simulink model "SYSTEM"  (R2026a)
settings: Solver=VariableStepAuto
model workspace (MAT data in the model file):
  CompAir_P : Simulink.ConnectionBus (value not decoded)
  CompAir_S : Simulink.Bus (value not decoded)
  Control_P : Simulink.ConnectionBus (value not decoded)
  Control_S : Simulink.Bus (value not decoded)
  CoolingFW_P : Simulink.ConnectionBus (value not decoded)
  CoolingFW_S : Simulink.Bus (value not decoded)
  FuelOil_P : Simulink.ConnectionBus (value not decoded)
  FuelOil_S : Simulink.Bus (value not decoded)
  Heat_P : Simulink.ConnectionBus (value not decoded)
  Heat_S : Simulink.Bus (value not decoded)
  LubeOil_P : Simulink.ConnectionBus (value not decoded)
  LubeOil_S : Simulink.Bus (value not decoded)
  Physical : Simulink.ConnectionBus (value not decoded)
  Power_P : Simulink.ConnectionBus (value not decoded)
  Power_S : Simulink.Bus (value not decoded)
  SaltWater_P : Simulink.ConnectionBus (value not decoded)
  SaltWater_S : Simulink.Bus (value not decoded)
  WasteGas_P : Simulink.ConnectionBus (value not decoded)
  WasteGas_S : Simulink.Bus (value not decoded)
  WasteOil_P : Simulink.ConnectionBus (value not decoded)
  WasteOil_S : Simulink.Bus (value not decoded)
  WasteSolid_P : Simulink.ConnectionBus (value not decoded)
  WasteSolid_S : Simulink.Bus (value not decoded)
  WasteWater_P : Simulink.ConnectionBus (value not decoded)
  WasteWater_S : Simulink.Bus (value not decoded)
undefined symbols (not defined in the file): FUEL
(part 5 of 5)

== system SYSTEM/SHIP/200 (PROPULSION)/21X (PROPULSORS)/21X WATER JET + MANEUVERING THRUSTER ==
  Bus Element In1 : Inport  PortName=42X-21XC
  Bus Element In3 : Inport  Port=2  PortName=51X-21XLO
  Bus Element In4 : Inport  Port=3  PortName=53X-21XCA
  Bus Element In2 : Inport  Port=4  PortName=50X-21XCFW
  10X-21X : PMIOPort  Side=Right  ConnectionType=Bus: Physical
  FROM 22X : PMIOPort  Port=2  Side=Right  ConnectionType=Bus: Physical
  Bus Element Out1 : Outport  PortName=21X-42XC
  Bus Element Out3 : Outport  Port=2  PortName=21X-51XLO
  Bus Element Out4 : Outport  Port=3  PortName=21X-53XCA
  Bus Element Out2 : Outport  Port=4  PortName=21X-50XCFW

== system SYSTEM/SHIP/200 (PROPULSION)/22X (SHAFTING)/22X ABSENT ==

== system SYSTEM/SHIP/200 (PROPULSION)/22X (SHAFTING)/22X MECHANICAL ==
  Bus Element In1 : Inport  PortName=51X-22XLO
  Bus Element In2 : Inport  Port=2  PortName=53X-22XCA
  TOFROM 23X : PMIOPort  Side=Right  ConnectionType=Bus: Physical
  10X-22X : PMIOPort  Port=2  Side=Right  ConnectionType=Bus: Physical
  TO 21X : PMIOPort  Port=3  Side=Right  ConnectionType=Bus: Physical
  Bus Element Out2 : Outport  PortName=22X-51XLO
  Bus Element Out3 : Outport  Port=2  PortName=22X-53XCA
  Bus Element Out1 : Outport  Port=3  PortName=22X-42XC

== system SYSTEM/SHIP/200 (PROPULSION)/23X (POWER TRANSMISSION)/23X ABSENT ==

== system SYSTEM/SHIP/200 (PROPULSION)/23X (POWER TRANSMISSION)/23X MECHANICAL ==
  Bus Element In2 : Inport  PortName=51X-23XLO
  Bus Element In1 : Inport  Port=2  PortName=42X-23XC
  TOFROM 22X : PMIOPort  Side=Left  ConnectionType=Bus: Physical
  FROM 20X : PMIOPort  Port=2  Side=Left  ConnectionType=Bus: Physical
  10X-23X : PMIOPort  Port=3  Side=Right  ConnectionType=Bus: Physical
  Bus Element Out3 : Outport  PortName=23X-51XLO
  Bus Element Out2 : Outport  Port=2  PortName=23X-42XC
  Bus Element Out1 : Outport  Port=3  PortName=23X-31XP

== system SYSTEM/SHIP/200 (PROPULSION)/23X (POWER TRANSMISSION)/23X MECHANICAL WITH POWER TAKEOFF ==
  Bus Element In2 : Inport  PortName=51X-23XLO
  Bus Element In1 : Inport  Port=2  PortName=42X-23XC
  TOFROM 22X : PMIOPort  Side=Left  ConnectionType=Bus: Physical
  FROM 20X : PMIOPort  Port=2  Side=Left  ConnectionType=Bus: Physical
  10X-23X : PMIOPort  Port=3  Side=Right  ConnectionType=Bus: Physical
  Bus Element Out3 : Outport  PortName=23X-51XLO
  Bus Element Out2 : Outport  Port=2  PortName=23X-42XC
  Bus Element Out1 : Outport  Port=3  PortName=23X-31XP

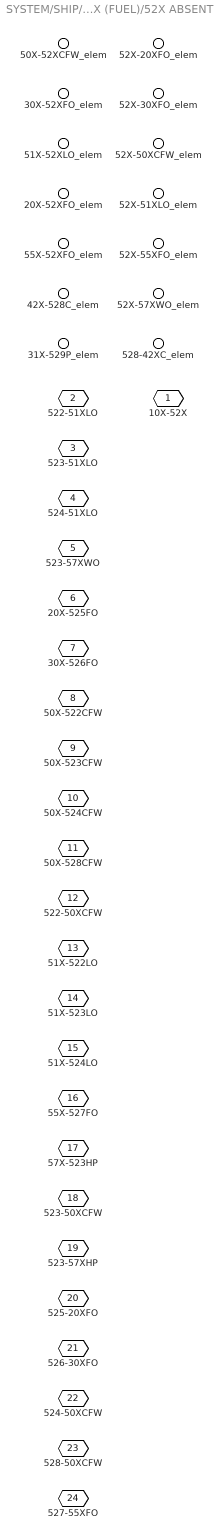
== system SYSTEM/SHIP/500 (AUXILLIARY SYSTEMS)/52X (FUEL)/52X ABSENT ==
  50X-52XCFW_elem : Inport  PortName=50X-52XCFW
  30X-52XFO_elem : Inport  Port=2  PortName=30X-52XFO
  51X-52XLO_elem : Inport  Port=3  PortName=51X-52XLO
  20X-52XFO_elem : Inport  Port=4  PortName=20X-52XFO
  55X-52XFO_elem : Inport  Port=5  PortName=55X-52XFO
  42X-528C_elem : Inport  Port=6  PortName=42X-528C
  31X-529P_elem : Inport  Port=7  PortName=31X-529P
  10X-52X : PMIOPort  Side=Right
  522-51XLO : PMIOPort  Port=2  Side=Left  ConnectionType=Bus: LubeOil_P
  523-51XLO : PMIOPort  Port=3  Side=Left  ConnectionType=Bus: LubeOil_P
  524-51XLO : PMIOPort  Port=4  Side=Left  ConnectionType=Bus: LubeOil_P
  523-57XWO : PMIOPort  Port=5  Side=Left  ConnectionType=Bus: WasteOil_P
  20X-525FO : PMIOPort  Port=6  Side=Left  ConnectionType=Bus: FuelOil_P
  30X-526FO : PMIOPort  Port=7  Side=Left  ConnectionType=Bus: FuelOil_P
  50X-522CFW : PMIOPort  Port=8  Side=Left  ConnectionType=Bus: CoolingFW_P
  50X-523CFW : PMIOPort  Port=9  Side=Left  ConnectionType=Bus: CoolingFW_P
  50X-524CFW : PMIOPort  Port=10  Side=Left  ConnectionType=Bus: CoolingFW_P
  50X-528CFW : PMIOPort  Port=11  Side=Left  ConnectionType=Bus: CoolingFW_P
  522-50XCFW : PMIOPort  Port=12  Side=Left  ConnectionType=Bus: CoolingFW_P
  51X-522LO : PMIOPort  Port=13  Side=Left  ConnectionType=Bus: LubeOil_P
  51X-523LO : PMIOPort  Port=14  Side=Left  ConnectionType=Bus: LubeOil_P
  51X-524LO : PMIOPort  Port=15  Side=Left  ConnectionType=Bus: LubeOil_P
  55X-527FO : PMIOPort  Port=16  Side=Left  ConnectionType=Bus: FuelOil_P
  57X-523HP : PMIOPort  Port=17  Side=Left  ConnectionType=Bus: Heat_P
  523-50XCFW : PMIOPort  Port=18  Side=Left  ConnectionType=Bus: CoolingFW_P
  523-57XHP : PMIOPort  Port=19  Side=Left  ConnectionType=Bus: Heat_P
  525-20XFO : PMIOPort  Port=20  Side=Left  ConnectionType=Bus: FuelOil_P
  526-30XFO : PMIOPort  Port=21  Side=Left  ConnectionType=Bus: FuelOil_P
  524-50XCFW : PMIOPort  Port=22  Side=Left  ConnectionType=Bus: CoolingFW_P
  528-50XCFW : PMIOPort  Port=23  Side=Left  ConnectionType=Bus: CoolingFW_P
  527-55XFO : PMIOPort  Port=24  Side=Left  ConnectionType=Bus: FuelOil_P
  52X-20XFO_elem : Outport  PortName=52X-20XFO
  52X-30XFO_elem : Outport  Port=2  PortName=52X-30XFO
  52X-50XCFW_elem : Outport  Port=3  PortName=52X-50XCFW
  52X-51XLO_elem : Outport  Port=4  PortName=52X-51XLO
  52X-55XFO_elem : Outport  Port=5  PortName=52X-55XFO
  52X-57XWO_elem : Outport  Port=6  PortName=52X-57XWO
  528-42XC_elem : Outport  Port=7  PortName=528-42XC

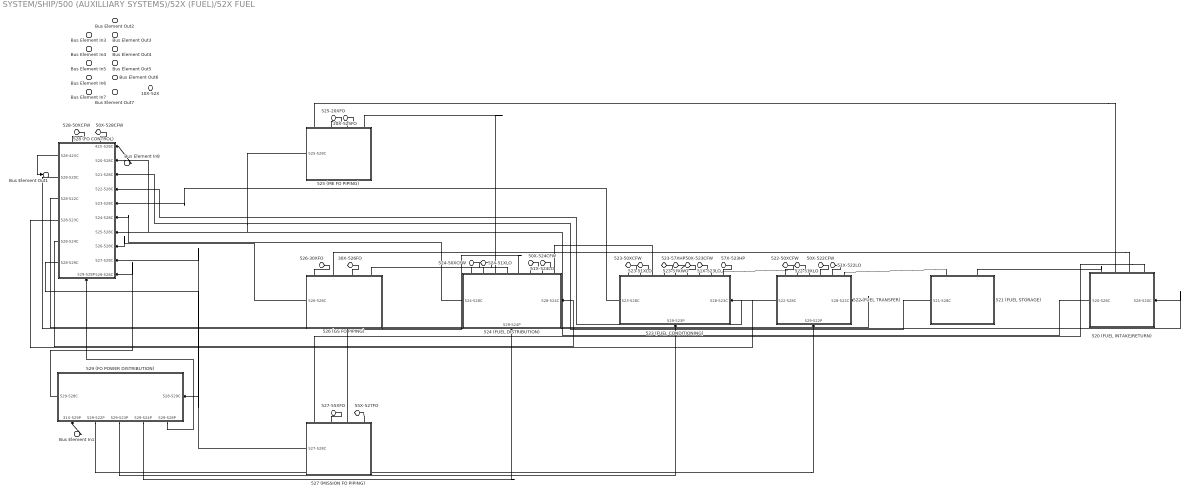
== system SYSTEM/SHIP/500 (AUXILLIARY SYSTEMS)/52X (FUEL)/52X FUEL ==
  Bus Element In3 : Inport  PortName=50X-52XCFW
  Bus Element In6 : Inport  Port=2  PortName=30X-52XFO
  Bus Element In4 : Inport  Port=3  PortName=51X-52XLO
  Bus Element In5 : Inport  Port=4  PortName=20X-52XFO
  Bus Element In7 : Inport  Port=5  PortName=55X-52XFO
  Bus Element In8 : Inport  Port=6  PortName=42X-528C
  Bus Element In1 : Inport  Port=7  PortName=31X-529P
  520 (FUEL INTAKE/RETURN) : Subsystem
      settings: PortSchema="{\"entries\":[{\"content\":{\"headerSize\":26,\"margin\":15,\"minimumSpacing\":25,\"sides\":[{\"content\":{\"connectorIds\":[\"Out1\"]},\"type\":\"ConnectorPlacement.EquallySpacedRectSide\",\"uuid\":\"4cfdffe2-3a28-4674-9aac-ff2f96812f2a\"},{\"content\":{\"connectorIds\":[\"In1\"],\"side\":\"RIGHT\"},\"type\":\"ConnectorPlacement.EquallySpacedRectSide\",\"uuid\":\"6bc321b8-6efb-4233-b1c1-d1363ffaceac\"},{\"content\":{\"connectorIds\":[\"LConn1\",\"RConn1\",\"RConn2\",\"RConn3\"],\"side\":\"TOP\"},\"type\":\"ConnectorPlacement.EquallySpacedRectSide\",\"uuid\":\"5128f762-77ab-4823-b460-d8c60ef20dad\"}]},\"type\":\"ConnectorPlacement.EquallySpacedConnector\",\"uuid\":\"2fe14ae3-6aef-4ed5-a4dc-a282704d28f8\"}],\"packageUris\":[\"http://schema.mathworks.com/mf0/Connector/R2020b\"],\"version\":\"1.0\"}"
  521 (FUEL STORAGE) : Subsystem
      settings: PortSchema="{\"entries\":[{\"content\":{\"headerSize\":26,\"margin\":15,\"minimumSpacing\":25,\"sides\":[{\"content\":{\"connectorIds\":[\"Out1\"]},\"type\":\"ConnectorPlacement.EquallySpacedRectSide\",\"uuid\":\"4cfdffe2-3a28-4674-9aac-ff2f96812f2a\"},{\"content\":{\"side\":\"RIGHT\"},\"type\":\"ConnectorPlacement.EquallySpacedRectSide\",\"uuid\":\"6bc321b8-6efb-4233-b1c1-d1363ffaceac\"},{\"content\":{\"connectorIds\":[\"LConn1\",\"RConn1\"],\"side\":\"TOP\"},\"type\":\"ConnectorPlacement.EquallySpacedRectSide\",\"uuid\":\"5128f762-77ab-4823-b460-d8c60ef20dad\"}]},\"type\":\"ConnectorPlacement.EquallySpacedConnector\",\"uuid\":\"2fe14ae3-6aef-4ed5-a4dc-a282704d28f8\"}],\"packageUris\":[\"http://schema.mathworks.com/mf0/Connector/R2020b\"],\"version\":\"1.0\"}"
  522 (FUEL TRANSFER) : Subsystem
      settings: PortSchema="{\"entries\":[{\"content\":{\"headerSize\":26,\"margin\":15,\"minimumSpacing\":25,\"sides\":[{\"content\":{\"connectorIds\":[\"Out1\"]},\"type\":\"ConnectorPlacement.EquallySpacedRectSide\",\"uuid\":\"4cfdffe2-3a28-4674-9aac-ff2f96812f2a\"},{\"content\":{\"connectorIds\":[\"In2\"],\"side\":\"RIGHT\"},\"type\":\"ConnectorPlacement.EquallySpacedRectSide\",\"uuid\":\"6bc321b8-6efb-4233-b1c1-d1363ffaceac\"},{\"content\":{\"connectorIds\":[\"LConn3\",\"LConn2\",\"LConn1\",\"LConn4\",\"LConn5\",\"RConn1\"],\"side\":\"TOP\"},\"type\":\"ConnectorPlacement.EquallySpacedRectSide\",\"uuid\":\"5128f762-77ab-4823-b460-d8c60ef20dad\"},{\"content\":{\"connectorIds\":[\"In1\"],\"side\":\"BOTTOM\"},\"type\":\"ConnectorPlacement.EquallySpacedRectSide\",\"uuid\":\"2a930d33-7a6a-4e0b-9580-44c950610589\"}]},\"type\":\"ConnectorPlacement.EquallySpacedConnector\",\"uuid\":\"2fe14ae3-6aef-4ed5-a4dc-a282704d28f8\"}],\"packageUris\":[\"http://schema.mathworks.com/mf0/Connector/R2020b\"],\"version\":\"1.0\"}"
  523 (FUEL CONDITIONING) : Subsystem
      settings: PortSchema="{\"entries\":[{\"content\":{\"headerSize\":26,\"margin\":15,\"minimumSpacing\":25,\"sides\":[{\"content\":{\"connectorIds\":[\"Out1\"]},\"type\":\"ConnectorPlacement.EquallySpacedRectSide\",\"uuid\":\"4cfdffe2-3a28-4674-9aac-ff2f96812f2a\"},{\"content\":{\"connectorIds\":[\"In2\"],\"side\":\"RIGHT\"},\"type\":\"ConnectorPlacement.EquallySpacedRectSide\",\"uuid\":\"6bc321b8-6efb-4233-b1c1-d1363ffaceac\"},{\"content\":{\"connectorIds\":[\"LConn3\",\"LConn2\",\"LConn1\",\"RConn2\",\"LConn4\",\"LConn5\",\"LConn6\",\"RConn3\",\"RConn1\"],\"side\":\"TOP\"},\"type\":\"ConnectorPlacement.EquallySpacedRectSide\",\"uuid\":\"5128f762-77ab-4823-b460-d8c60ef20dad\"},{\"content\":{\"connectorIds\":[\"In1\"],\"side\":\"BOTTOM\"},\"type\":\"ConnectorPlacement.EquallySpacedRectSide\",\"uuid\":\"0a36b159-1b21-43db-be33-33362cd12218\"}]},\"type\":\"ConnectorPlacement.EquallySpacedConnector\",\"uuid\":\"2fe14ae3-6aef-4ed5-a4dc-a282704d28f8\"}],\"packageUris\":[\"http://schema.mathworks.com/mf0/Connector/R2020b\"],\"version\":\"1.0\"}"
  524 (FUEL DISTRIBUTION) : Subsystem
      settings: PortSchema="{\"entries\":[{\"content\":{\"headerSize\":26,\"margin\":15,\"minimumSpacing\":25,\"sides\":[{\"content\":{\"connectorIds\":[\"Out1\"]},\"type\":\"ConnectorPlacement.EquallySpacedRectSide\",\"uuid\":\"4cfdffe2-3a28-4674-9aac-ff2f96812f2a\"},{\"content\":{\"connectorIds\":[\"In2\"],\"side\":\"RIGHT\"},\"type\":\"ConnectorPlacement.EquallySpacedRectSide\",\"uuid\":\"6bc321b8-6efb-4233-b1c1-d1363ffaceac\"},{\"content\":{\"connectorIds\":[\"LConn5\",\"LConn2\",\"LConn1\",\"LConn3\",\"LConn4\",\"LConn6\",\"LConn7\",\"RConn1\"],\"side\":\"TOP\"},\"type\":\"ConnectorPlacement.EquallySpacedRectSide\",\"uuid\":\"5128f762-77ab-4823-b460-d8c60ef20dad\"},{\"content\":{\"connectorIds\":[\"In1\"],\"side\":\"BOTTOM\"},\"type\":\"ConnectorPlacement.EquallySpacedRectSide\",\"uuid\":\"af17bfb2-26c0-4d79-9f41-99ac55d94094\"}]},\"type\":\"ConnectorPlacement.EquallySpacedConnector\",\"uuid\":\"2fe14ae3-6aef-4ed5-a4dc-a282704d28f8\"}],\"packageUris\":[\"http://schema.mathworks.com/mf0/Connector/R2020b\"],\"version\":\"1.0\"}"
  525 (ME FO PIPING) : Subsystem  Variant=on  VariantControlMode=label  LabelModeActiveChoice=525 (ME FO PIPING)
      settings: PortSchema="{\"entries\":[{\"content\":{\"headerSize\":38,\"margin\":15,\"minimumSpacing\":25,\"sides\":[{\"content\":{\"connectorIds\":[\"Out1\"]},\"type\":\"ConnectorPlacement.EquallySpacedRectSide\",\"uuid\":\"4cfdffe2-3a28-4674-9aac-ff2f96812f2a\"},{\"content\":{\"side\":\"RIGHT\"},\"type\":\"ConnectorPlacement.EquallySpacedRectSide\",\"uuid\":\"6bc321b8-6efb-4233-b1c1-d1363ffaceac\"},{\"content\":{\"connectorIds\":[\"LConn1\",\"LConn2\",\"RConn2\",\"RConn1\"],\"side\":\"TOP\"},\"type\":\"ConnectorPlacement.EquallySpacedRectSide\",\"uuid\":\"5128f762-77ab-4823-b460-d8c60ef20dad\"}]},\"type\":\"ConnectorPlacement.EquallySpacedConnector\",\"uuid\":\"2fe14ae3-6aef-4ed5-a4dc-a282704d28f8\"}],\"packageUris\":[\"http://schema.mathworks.com/mf0/Connector/R2020b\"],\"version\":\"1.0\"}"
  526 (GS FO PIPING) : Subsystem  Variant=on  VariantControlMode=label  LabelModeActiveChoice=526 (GS FO PIPING)
      settings: PortSchema="{\"entries\":[{\"content\":{\"headerSize\":38,\"margin\":15,\"minimumSpacing\":25,\"sides\":[{\"content\":{\"connectorIds\":[\"Out1\"]},\"type\":\"ConnectorPlacement.EquallySpacedRectSide\",\"uuid\":\"4cfdffe2-3a28-4674-9aac-ff2f96812f2a\"},{\"content\":{\"side\":\"RIGHT\"},\"type\":\"ConnectorPlacement.EquallySpacedRectSide\",\"uuid\":\"6bc321b8-6efb-4233-b1c1-d1363ffaceac\"},{\"content\":{\"connectorIds\":[\"LConn2\",\"LConn1\",\"RConn2\",\"RConn1\"],\"side\":\"TOP\"},\"type\":\"ConnectorPlacement.EquallySpacedRectSide\",\"uuid\":\"5128f762-77ab-4823-b460-d8c60ef20dad\"}]},\"type\":\"ConnectorPlacement.EquallySpacedConnector\",\"uuid\":\"2fe14ae3-6aef-4ed5-a4dc-a282704d28f8\"}],\"packageUris\":[\"http://schema.mathworks.com/mf0/Connector/R2020b\"],\"version\":\"1.0\"}"
  527 (MISSION FO PIPING) : Subsystem  Variant=on  VariantControlMode=label  LabelModeActiveChoice=527 (MISSION FO PIPING)
      settings: PortSchema="{\"entries\":[{\"content\":{\"headerSize\":38,\"margin\":15,\"minimumSpacing\":25,\"sides\":[{\"content\":{\"connectorIds\":[\"Out1\"]},\"type\":\"ConnectorPlacement.EquallySpacedRectSide\",\"uuid\":\"4cfdffe2-3a28-4674-9aac-ff2f96812f2a\"},{\"content\":{\"side\":\"RIGHT\"},\"type\":\"ConnectorPlacement.EquallySpacedRectSide\",\"uuid\":\"6bc321b8-6efb-4233-b1c1-d1363ffaceac\"},{\"content\":{\"connectorIds\":[\"LConn1\",\"LConn2\",\"RConn1\",\"RConn2\"],\"side\":\"TOP\"},\"type\":\"ConnectorPlacement.EquallySpacedRectSide\",\"uuid\":\"5128f762-77ab-4823-b460-d8c60ef20dad\"}]},\"type\":\"ConnectorPlacement.EquallySpacedConnector\",\"uuid\":\"2fe14ae3-6aef-4ed5-a4dc-a282704d28f8\"}],\"packageUris\":[\"http://schema.mathworks.com/mf0/Connector/R2020b\"],\"version\":\"1.0\"}"
  528 (FO CONTROL) : Subsystem
      settings: PortSchema="{\"entries\":[{\"content\":{\"headerSize\":26,\"margin\":15,\"minimumSpacing\":25,\"sides\":[{\"content\":{\"connectorIds\":[\"Out1\",\"Out2\",\"Out3\",\"Out4\",\"Out5\",\"Out6\"]},\"type\":\"ConnectorPlacement.EquallySpacedRectSide\",\"uuid\":\"4cfdffe2-3a28-4674-9aac-ff2f96812f2a\"},{\"content\":{\"connectorIds\":[\"In2\",\"In3\",\"In4\",\"In5\",\"In6\",\"In7\",\"In8\",\"In9\",\"In10\",\"In11\"],\"side\":\"RIGHT\"},\"type\":\"ConnectorPlacement.EquallySpacedRectSide\",\"uuid\":\"6bc321b8-6efb-4233-b1c1-d1363ffaceac\"},{\"content\":{\"connectorIds\":[\"LConn1\",\"LConn2\"],\"side\":\"TOP\"},\"type\":\"ConnectorPlacement.EquallySpacedRectSide\",\"uuid\":\"5128f762-77ab-4823-b460-d8c60ef20dad\"},{\"content\":{\"connectorIds\":[\"In1\"],\"side\":\"BOTTOM\"},\"type\":\"ConnectorPlacement.EquallySpacedRectSide\",\"uuid\":\"be85725a-6fe0-4fb4-958b-07653a845403\"}]},\"type\":\"ConnectorPlacement.EquallySpacedConnector\",\"uuid\":\"2fe14ae3-6aef-4ed5-a4dc-a282704d28f8\"}],\"packageUris\":[\"http://schema.mathworks.com/mf0/Connector/R2020b\"],\"version\":\"1.0\"}"
  529 (FO POWER DISTRIBUTION) : Subsystem
      settings: PortSchema="{\"entries\":[{\"content\":{\"headerSize\":26,\"margin\":15,\"minimumSpacing\":25,\"sides\":[{\"content\":{\"connectorIds\":[\"Out5\"]},\"type\":\"ConnectorPlacement.EquallySpacedRectSide\",\"uuid\":\"4cfdffe2-3a28-4674-9aac-ff2f96812f2a\"},{\"content\":{\"connectorIds\":[\"In2\"],\"side\":\"RIGHT\"},\"type\":\"ConnectorPlacement.EquallySpacedRectSide\",\"uuid\":\"6bc321b8-6efb-4233-b1c1-d1363ffaceac\"},{\"content\":{\"side\":\"TOP\"},\"type\":\"ConnectorPlacement.EquallySpacedRectSide\",\"uuid\":\"5128f762-77ab-4823-b460-d8c60ef20dad\"},{\"content\":{\"connectorIds\":[\"In1\",\"Out1\",\"Out2\",\"Out3\",\"Out4\"],\"side\":\"BOTTOM\"},\"type\":\"ConnectorPlacement.EquallySpacedRectSide\",\"uuid\":\"48bb8438-8d1f-4b5d-82c5-6a5b54cc9ed4\"}]},\"type\":\"ConnectorPlacement.EquallySpacedConnector\",\"uuid\":\"2fe14ae3-6aef-4ed5-a4dc-a282704d28f8\"}],\"packageUris\":[\"http://schema.mathworks.com/mf0/Connector/R2020b\"],\"version\":\"1.0\"}"
  10X-52X : PMIOPort  Side=Right  ConnectionType=Bus: Physical
  522-50XCFW : PMIOPort  Port=2  Side=Left  ConnectionType=Bus: CoolingFW_P
  523-50XCFW : PMIOPort  Port=3  Side=Left  ConnectionType=Bus: CoolingFW_P
  523-57XHP : PMIOPort  Port=4  Side=Left  ConnectionType=Bus: Heat_P
  525-20XFO : PMIOPort  Port=5  Side=Left  ConnectionType=Bus: FuelOil_P
  526-30XFO : PMIOPort  Port=6  Side=Left  ConnectionType=Bus: FuelOil_P
  524-50XCFW : PMIOPort  Port=7  Side=Left  ConnectionType=Bus: CoolingFW_P
  528-50XCFW : PMIOPort  Port=8  Side=Left  ConnectionType=Bus: CoolingFW_P
  527-55XFO : PMIOPort  Port=9  Side=Left  ConnectionType=Bus: FuelOil_P
  522-51XLO : PMIOPort  Port=10  Side=Left  ConnectionType=Bus: LubeOil_P
  523-51XLO : PMIOPort  Port=11  Side=Left  ConnectionType=Bus: LubeOil_P
  524-51XLO : PMIOPort  Port=12  Side=Left  ConnectionType=Bus: LubeOil_P
  523-57XWO : PMIOPort  Port=13  Side=Left  ConnectionType=Bus: WasteOil_P
  20X-525FO : PMIOPort  Port=14  Side=Left  ConnectionType=Bus: FuelOil_P
  30X-526FO : PMIOPort  Port=15  Side=Left  ConnectionType=Bus: FuelOil_P
  50X-522CFW : PMIOPort  Port=16  Side=Left  ConnectionType=Bus: CoolingFW_P
  50X-523CFW : PMIOPort  Port=17  Side=Left  ConnectionType=Bus: CoolingFW_P
  50X-524CFW : PMIOPort  Port=18  Side=Left  ConnectionType=Bus: CoolingFW_P
  50X-528CFW : PMIOPort  Port=19  Side=Left  ConnectionType=Bus: CoolingFW_P
  51X-522LO : PMIOPort  Port=20  Side=Left  ConnectionType=Bus: LubeOil_P
  51X-523LO : PMIOPort  Port=21  Side=Left  ConnectionType=Bus: LubeOil_P
  51X-524LO : PMIOPort  Port=22  Side=Left  ConnectionType=Bus: LubeOil_P
  55X-527FO : PMIOPort  Port=23  Side=Left  ConnectionType=Bus: FuelOil_P
  57X-523HP : PMIOPort  Port=24  Side=Left  ConnectionType=Bus: Heat_P
  Bus Element Out4 : Outport  PortName=52X-20XFO
  Bus Element Out5 : Outport  Port=2  PortName=52X-30XFO
  Bus Element Out2 : Outport  Port=3  PortName=52X-50XCFW
  Bus Element Out3 : Outport  Port=4  PortName=52X-51XLO
  Bus Element Out6 : Outport  Port=5  PortName=52X-55XFO
  Bus Element Out7 : Outport  Port=6  PortName=52X-57XWO
  Bus Element Out1 : Outport  Port=7  PortName=528-42XC
  wires:
  Bus Element In8/1 -> 528 (FO CONTROL)/2(42X-528C)
  528 (FO CONTROL)/1(528-42XC) -> Bus Element Out1/1
  528 (FO CONTROL)/2(528-520C) -> 520 (FUEL INTAKE/RETURN)/1(528-520C)
  528 (FO CONTROL)/3(528-522C) -> 522 (FUEL TRANSFER)/2(528-522C)
  528 (FO CONTROL)/4(528-523C) -> 523 (FUEL CONDITIONING)/2(528-523C)
  528 (FO CONTROL)/5(528-524C) -> 524 (FUEL DISTRIBUTION)/2(528-524C)
  520 (FUEL INTAKE/RETURN)/1(520-528C) -> 528 (FO CONTROL)/3(520-528C)
  521 (FUEL STORAGE)/1(521-528C) -> 528 (FO CONTROL)/4(521-528C)
  522 (FUEL TRANSFER)/1(522-528C) -> 528 (FO CONTROL)/5(522-528C)
  523 (FUEL CONDITIONING)/1(523-528C) -> 528 (FO CONTROL)/6(523-528C)
  524 (FUEL DISTRIBUTION)/1(524-528C) -> 528 (FO CONTROL)/7(524-528C)
  529 (FO POWER DISTRIBUTION)/5(529-528C) -> 528 (FO CONTROL)/11(529-528C)
  528 (FO CONTROL)/6(528-529C) -> 529 (FO POWER DISTRIBUTION)/2(528-529C)
  Bus Element In1/1 -> 529 (FO POWER DISTRIBUTION)/1(31X-529P)
  529 (FO POWER DISTRIBUTION)/4(529-528P) -> 528 (FO CONTROL)/1(529-528P)
  529 (FO POWER DISTRIBUTION)/3(529-524P) -> 524 (FUEL DISTRIBUTION)/1(529-524P)
  529 (FO POWER DISTRIBUTION)/2(529-523P) -> 523 (FUEL CONDITIONING)/1(529-523P)
  529 (FO POWER DISTRIBUTION)/1(529-522P) -> 522 (FUEL TRANSFER)/1(529-522P)
  525 (ME FO PIPING)/1(525-528C) -> 528 (FO CONTROL)/8(525-528C)
  526 (GS FO PIPING)/1(526-528C) -> 528 (FO CONTROL)/9(526-528C)
  527 (MISSION FO PIPING)/1(527-528C) -> 528 (FO CONTROL)/10(527-528C)
  connections:
  520 (FUEL INTAKE/RETURN)/LConn1 -- 521 (FUEL STORAGE)/RConn1
  521 (FUEL STORAGE)/LConn1 -- 522 (FUEL TRANSFER)/RConn1
  522 (FUEL TRANSFER)/LConn1 -- 523 (FUEL CONDITIONING)/RConn3
  523 (FUEL CONDITIONING)/LConn1 -- 524 (FUEL DISTRIBUTION)/RConn1
  523 (FUEL CONDITIONING)/RConn1 -- 57X-523HP/RConn1
  523 (FUEL CONDITIONING)/RConn2 -- 523-57XHP/RConn1
  528 (FO CONTROL)/LConn1 -- 528-50XCFW/RConn1
  524 (FUEL DISTRIBUTION)/LConn5 -- 524-50XCFW/RConn1
  528 (FO CONTROL)/LConn2 -- 50X-528CFW/RConn1
  522 (FUEL TRANSFER)/LConn4 -- 50X-522CFW/RConn1
  523 (FUEL CONDITIONING)/LConn5 -- 50X-523CFW/RConn1
  524 (FUEL DISTRIBUTION)/LConn6 -- 50X-524CFW/RConn1
  522 (FUEL TRANSFER)/LConn3 -- 522-50XCFW/RConn1
  523 (FUEL CONDITIONING)/LConn3 -- 523-50XCFW/RConn1
  524 (FUEL DISTRIBUTION)/LConn2 -- 524-51XLO/RConn1
  523 (FUEL CONDITIONING)/LConn2 -- 523-51XLO/RConn1
  522 (FUEL TRANSFER)/LConn2 -- 522-51XLO/RConn1
  522 (FUEL TRANSFER)/LConn5 -- 51X-522LO/RConn1
  523 (FUEL CONDITIONING)/LConn6 -- 51X-523LO/RConn1
  524 (FUEL DISTRIBUTION)/LConn7 -- 51X-524LO/RConn1
  523-57XWO/RConn1 -- 523 (FUEL CONDITIONING)/LConn4
  525 (ME FO PIPING)/LConn1 -- 520 (FUEL INTAKE/RETURN)/RConn1
  525 (ME FO PIPING)/LConn2 -- 525-20XFO/RConn1
  525 (ME FO PIPING)/RConn1 -- 524 (FUEL DISTRIBUTION)/LConn1
  525 (ME FO PIPING)/RConn2 -- 20X-525FO/RConn1
  526 (GS FO PIPING)/LConn1 -- 520 (FUEL INTAKE/RETURN)/RConn2
  526 (GS FO PIPING)/LConn2 -- 526-30XFO/RConn1
  526 (GS FO PIPING)/RConn1 -- 524 (FUEL DISTRIBUTION)/LConn3
  526 (GS FO PIPING)/RConn2 -- 30X-526FO/RConn1
  527 (MISSION FO PIPING)/LConn1 -- 520 (FUEL INTAKE/RETURN)/RConn3
  527 (MISSION FO PIPING)/LConn2 -- 527-55XFO/RConn1
  527 (MISSION FO PIPING)/RConn1 -- 524 (FUEL DISTRIBUTION)/LConn4
  527 (MISSION FO PIPING)/RConn2 -- 55X-527FO/RConn1

== system SYSTEM/SHIP/500 (AUXILLIARY SYSTEMS)/52X (FUEL)/52X FUEL/520 (FUEL INTAKE//RETURN) ==
  Bus Element In1 : Inport  PortName=528-520C
  520-521FO : PMIOPort  Side=Left  ConnectionType=Bus: FuelOil_P
  525-520FO : PMIOPort  Port=2  Side=Right  ConnectionType=Bus: FuelOil_P
  526-520FO : PMIOPort  Port=3  Side=Right  ConnectionType=Bus: FuelOil_P
  527-520FO : PMIOPort  Port=4  Side=Right  ConnectionType=Bus: FuelOil_P
  Bus Element Out1 : Outport  PortName=520-528C

== system SYSTEM/SHIP/500 (AUXILLIARY SYSTEMS)/52X (FUEL)/52X FUEL/521 (FUEL STORAGE) ==
  520-521FO : PMIOPort  Side=Right  ConnectionType=Bus: FuelOil_P
  521-522FO : PMIOPort  Port=2  Side=Left  ConnectionType=Bus: FuelOil_P
  Bus Element Out1 : Outport  PortName=521-528C

== system SYSTEM/SHIP/500 (AUXILLIARY SYSTEMS)/52X (FUEL)/52X FUEL/522 (FUEL TRANSFER) ==
  Bus Element In2 : Inport  PortName=529-522P
  Bus Element In1 : Inport  Port=2  PortName=528-522C
  521-522FO : PMIOPort  Side=Right  ConnectionType=Bus: FuelOil_P
  522-523FO : PMIOPort  Port=2  Side=Left  ConnectionType=Bus: FuelOil_P
  522-51XLO : PMIOPort  Port=3  Side=Left  ConnectionType=Bus: LubeOil_P
  522-50XCFW : PMIOPort  Port=4  Side=Left  ConnectionType=Bus: CoolingFW_P
  50X-522CFW : PMIOPort  Port=5  Side=Left  ConnectionType=Bus: CoolingFW_P
  51X-522LO : PMIOPort  Port=6  Side=Left  ConnectionType=Bus: LubeOil_P
  Bus Element Out1 : Outport  PortName=522-528C

== system SYSTEM/SHIP/500 (AUXILLIARY SYSTEMS)/52X (FUEL)/52X FUEL/523 (FUEL CONDITIONING) ==
  Bus Element In2 : Inport  PortName=529-523P
  Bus Element In1 : Inport  Port=2  PortName=528-523C
  57X-523HP : PMIOPort  Side=Right  ConnectionType=Bus: Heat_P
  523-57XHP : PMIOPort  Port=2  Side=Right  ConnectionType=Bus: Heat_P
  522-523FO : PMIOPort  Port=3  Side=Right  ConnectionType=Bus: FuelOil_P
  523-524FO : PMIOPort  Port=4  Side=Left  ConnectionType=Bus: FuelOil_P
  523-51XLO : PMIOPort  Port=5  Side=Left  ConnectionType=Bus: LubeOil_P
  523-50XCFW : PMIOPort  Port=6  Side=Left  ConnectionType=Bus: CoolingFW_P
  523-57XWO : PMIOPort  Port=7  Side=Left  ConnectionType=Bus: WasteOil_P
  50X-523CFW : PMIOPort  Port=8  Side=Left  ConnectionType=Bus: CoolingFW_P
  51X-523LO : PMIOPort  Port=9  Side=Left  ConnectionType=Bus: LubeOil_P
  Bus Element Out1 : Outport  PortName=523-528C

== system SYSTEM/SHIP/500 (AUXILLIARY SYSTEMS)/52X (FUEL)/52X FUEL/524 (FUEL DISTRIBUTION) ==
  Bus Element In2 : Inport  PortName=529-524P
  Bus Element In1 : Inport  Port=2  PortName=528-524C
  523-524FO : PMIOPort  Side=Right  ConnectionType=Bus: FuelOil_P
  524-525FO : PMIOPort  Port=2  Side=Left  ConnectionType=Bus: FuelOil_P
  524-51XLO : PMIOPort  Port=3  Side=Left  ConnectionType=Bus: LubeOil_P
  524-526FO : PMIOPort  Port=4  Side=Left  ConnectionType=Bus: FuelOil_P
  524-527FO : PMIOPort  Port=5  Side=Left  ConnectionType=Bus: FuelOil_P
  524-50XCFW : PMIOPort  Port=6  Side=Left  ConnectionType=Bus: CoolingFW_P
  50X-524CFW : PMIOPort  Port=7  Side=Left  ConnectionType=Bus: CoolingFW_P
  51X-524LO : PMIOPort  Port=8  Side=Left  ConnectionType=Bus: LubeOil_P
  Bus Element Out1 : Outport  PortName=524-528C

== system SYSTEM/SHIP/500 (AUXILLIARY SYSTEMS)/52X (FUEL)/52X FUEL/525 (ME FO PIPING) ==
  525 ABSENT : Subsystem  VariantControl=525 ABSENT
      settings: PortSchema="{\"entries\":[{\"content\":{\"headerSize\":26,\"margin\":15,\"minimumSpacing\":25,\"sides\":[{\"content\":{\"connectorIds\":[\"Out1\"]},\"type\":\"ConnectorPlacement.EquallySpacedRectSide\",\"uuid\":\"4cfdffe2-3a28-4674-9aac-ff2f96812f2a\"},{\"content\":{\"side\":\"RIGHT\"},\"type\":\"ConnectorPlacement.EquallySpacedRectSide\",\"uuid\":\"6bc321b8-6efb-4233-b1c1-d1363ffaceac\"},{\"content\":{\"connectorIds\":[\"LConn1\",\"LConn2\",\"RConn2\",\"RConn1\"],\"side\":\"TOP\"},\"type\":\"ConnectorPlacement.EquallySpacedRectSide\",\"uuid\":\"5128f762-77ab-4823-b460-d8c60ef20dad\"}]},\"type\":\"ConnectorPlacement.EquallySpacedConnector\",\"uuid\":\"2fe14ae3-6aef-4ed5-a4dc-a282704d28f8\"}],\"packageUris\":[\"http://schema.mathworks.com/mf0/Connector/R2020b\"],\"version\":\"1.0\"}"
  525 ME FO PIPING : Subsystem  VariantControl=525 (ME FO PIPING)
      settings: PortSchema="{\"entries\":[{\"content\":{\"headerSize\":26,\"margin\":15,\"minimumSpacing\":25,\"sides\":[{\"content\":{\"connectorIds\":[\"Out1\"]},\"type\":\"ConnectorPlacement.EquallySpacedRectSide\",\"uuid\":\"4cfdffe2-3a28-4674-9aac-ff2f96812f2a\"},{\"content\":{\"side\":\"RIGHT\"},\"type\":\"ConnectorPlacement.EquallySpacedRectSide\",\"uuid\":\"6bc321b8-6efb-4233-b1c1-d1363ffaceac\"},{\"content\":{\"connectorIds\":[\"LConn1\",\"LConn2\",\"RConn2\",\"RConn1\"],\"side\":\"TOP\"},\"type\":\"ConnectorPlacement.EquallySpacedRectSide\",\"uuid\":\"5128f762-77ab-4823-b460-d8c60ef20dad\"}]},\"type\":\"ConnectorPlacement.EquallySpacedConnector\",\"uuid\":\"2fe14ae3-6aef-4ed5-a4dc-a282704d28f8\"}],\"packageUris\":[\"http://schema.mathworks.com/mf0/Connector/R2020b\"],\"version\":\"1.0\"}"
  524-525FO : PMIOPort  Side=Right  ConnectionType=Bus: FuelOil_P
  525-520FO : PMIOPort  Port=2  Side=Left  ConnectionType=Bus: FuelOil_P
  525-20XFO : PMIOPort  Port=3  Side=Left  ConnectionType=Bus: FuelOil_P
  20X-525FO : PMIOPort  Port=4  Side=Right  ConnectionType=Bus: FuelOil_P
  525-528C : Outport  OutDataTypeStr=Bus: Control_S

== system SYSTEM/SHIP/500 (AUXILLIARY SYSTEMS)/52X (FUEL)/52X FUEL/526 (GS FO PIPING) ==
  526 ABSENT : Subsystem  VariantControl=526 ABSENT
      settings: PortSchema="{\"entries\":[{\"content\":{\"headerSize\":26,\"margin\":15,\"minimumSpacing\":25,\"sides\":[{\"content\":{\"connectorIds\":[\"Out1\"]},\"type\":\"ConnectorPlacement.EquallySpacedRectSide\",\"uuid\":\"4cfdffe2-3a28-4674-9aac-ff2f96812f2a\"},{\"content\":{\"side\":\"RIGHT\"},\"type\":\"ConnectorPlacement.EquallySpacedRectSide\",\"uuid\":\"6bc321b8-6efb-4233-b1c1-d1363ffaceac\"},{\"content\":{\"connectorIds\":[\"LConn2\",\"LConn1\",\"RConn2\",\"RConn1\"],\"side\":\"TOP\"},\"type\":\"ConnectorPlacement.EquallySpacedRectSide\",\"uuid\":\"5128f762-77ab-4823-b460-d8c60ef20dad\"}]},\"type\":\"ConnectorPlacement.EquallySpacedConnector\",\"uuid\":\"2fe14ae3-6aef-4ed5-a4dc-a282704d28f8\"}],\"packageUris\":[\"http://schema.mathworks.com/mf0/Connector/R2020b\"],\"version\":\"1.0\"}"
  526 GS FO PIPING : Subsystem  VariantControl=526 (GS FO PIPING)
      settings: PortSchema="{\"entries\":[{\"content\":{\"headerSize\":26,\"margin\":15,\"minimumSpacing\":25,\"sides\":[{\"content\":{\"connectorIds\":[\"Out1\"]},\"type\":\"ConnectorPlacement.EquallySpacedRectSide\",\"uuid\":\"4cfdffe2-3a28-4674-9aac-ff2f96812f2a\"},{\"content\":{\"side\":\"RIGHT\"},\"type\":\"ConnectorPlacement.EquallySpacedRectSide\",\"uuid\":\"6bc321b8-6efb-4233-b1c1-d1363ffaceac\"},{\"content\":{\"connectorIds\":[\"LConn2\",\"LConn1\",\"RConn2\",\"RConn1\"],\"side\":\"TOP\"},\"type\":\"ConnectorPlacement.EquallySpacedRectSide\",\"uuid\":\"5128f762-77ab-4823-b460-d8c60ef20dad\"}]},\"type\":\"ConnectorPlacement.EquallySpacedConnector\",\"uuid\":\"2fe14ae3-6aef-4ed5-a4dc-a282704d28f8\"}],\"packageUris\":[\"http://schema.mathworks.com/mf0/Connector/R2020b\"],\"version\":\"1.0\"}"
  524-526FO : PMIOPort  Side=Right  ConnectionType=Bus: FuelOil_P
  526-520FO : PMIOPort  Port=2  Side=Left  ConnectionType=Bus: FuelOil_P
  526-30XFO : PMIOPort  Port=3  Side=Left  ConnectionType=Bus: FuelOil_P
  30X-526FO : PMIOPort  Port=4  Side=Right  ConnectionType=Bus: FuelOil_P
  526-528C : Outport  OutDataTypeStr=Bus: Control_S

== system SYSTEM/SHIP/500 (AUXILLIARY SYSTEMS)/52X (FUEL)/52X FUEL/527 (MISSION FO PIPING) ==
  527 ABSENT : Subsystem  VariantControl=527 ABSENT
      settings: PortSchema="{\"entries\":[{\"content\":{\"headerSize\":26,\"margin\":15,\"minimumSpacing\":25,\"sides\":[{\"content\":{\"connectorIds\":[\"Out1\"]},\"type\":\"ConnectorPlacement.EquallySpacedRectSide\",\"uuid\":\"4cfdffe2-3a28-4674-9aac-ff2f96812f2a\"},{\"content\":{\"side\":\"RIGHT\"},\"type\":\"ConnectorPlacement.EquallySpacedRectSide\",\"uuid\":\"6bc321b8-6efb-4233-b1c1-d1363ffaceac\"},{\"content\":{\"connectorIds\":[\"LConn1\",\"LConn2\",\"RConn1\",\"RConn2\"],\"side\":\"TOP\"},\"type\":\"ConnectorPlacement.EquallySpacedRectSide\",\"uuid\":\"5128f762-77ab-4823-b460-d8c60ef20dad\"}]},\"type\":\"ConnectorPlacement.EquallySpacedConnector\",\"uuid\":\"2fe14ae3-6aef-4ed5-a4dc-a282704d28f8\"}],\"packageUris\":[\"http://schema.mathworks.com/mf0/Connector/R2020b\"],\"version\":\"1.0\"}"
  527 MISSION FO PIPING : Subsystem  VariantControl=527 (MISSION FO PIPING)
      settings: PortSchema="{\"entries\":[{\"content\":{\"headerSize\":26,\"margin\":15,\"minimumSpacing\":25,\"sides\":[{\"content\":{\"connectorIds\":[\"Out1\"]},\"type\":\"ConnectorPlacement.EquallySpacedRectSide\",\"uuid\":\"4cfdffe2-3a28-4674-9aac-ff2f96812f2a\"},{\"content\":{\"side\":\"RIGHT\"},\"type\":\"ConnectorPlacement.EquallySpacedRectSide\",\"uuid\":\"6bc321b8-6efb-4233-b1c1-d1363ffaceac\"},{\"content\":{\"connectorIds\":[\"LConn1\",\"LConn2\",\"RConn1\",\"RConn2\"],\"side\":\"TOP\"},\"type\":\"ConnectorPlacement.EquallySpacedRectSide\",\"uuid\":\"5128f762-77ab-4823-b460-d8c60ef20dad\"}]},\"type\":\"ConnectorPlacement.EquallySpacedConnector\",\"uuid\":\"2fe14ae3-6aef-4ed5-a4dc-a282704d28f8\"}],\"packageUris\":[\"http://schema.mathworks.com/mf0/Connector/R2020b\"],\"version\":\"1.0\"}"
  524-527FO : PMIOPort  Side=Right  ConnectionType=Bus: FuelOil_P
  527-520FO : PMIOPort  Port=2  Side=Left  ConnectionType=Bus: FuelOil_P
  527-55XFO : PMIOPort  Port=3  Side=Left  ConnectionType=Bus: FuelOil_P
  55X-527FO : PMIOPort  Port=4  Side=Right  ConnectionType=Bus: FuelOil_P
  527-528C : Outport  OutDataTypeStr=Bus: Control_S

== system SYSTEM/SHIP/500 (AUXILLIARY SYSTEMS)/52X (FUEL)/52X FUEL/528 (FO CONTROL) ==
  Bus Element In11 : Inport  PortName=529-528P
  Bus Element In1 : Inport  Port=2  PortName=42X-528C
  Bus Element In2 : Inport  Port=3  PortName=520-528C
  Bus Element In3 : Inport  Port=4  PortName=521-528C
  Bus Element In4 : Inport  Port=5  PortName=522-528C
  Bus Element In5 : Inport  Port=6  PortName=523-528C
  Bus Element In6 : Inport  Port=7  PortName=524-528C
  Bus Element In7 : Inport  Port=8  PortName=525-528C
  Bus Element In8 : Inport  Port=9  PortName=526-528C
  Bus Element In9 : Inport  Port=10  PortName=527-528C
  Bus Element In10 : Inport  Port=11  PortName=529-528C
  528-50XCFW : PMIOPort  Side=Left  ConnectionType=Bus: CoolingFW_P
  50X-528CFW : PMIOPort  Port=2  Side=Left  ConnectionType=Bus: CoolingFW_P
  Bus Element Out1 : Outport  PortName=528-42XC
  Bus Element Out2 : Outport  Port=2  PortName=528-520C
  Bus Element Out3 : Outport  Port=3  PortName=528-522C
  Bus Element Out4 : Outport  Port=4  PortName=528-523C
  Bus Element Out5 : Outport  Port=5  PortName=528-524C
  Bus Element Out6 : Outport  Port=6  PortName=528-529C

== system SYSTEM/SHIP/500 (AUXILLIARY SYSTEMS)/52X (FUEL)/52X FUEL/529 (FO POWER DISTRIBUTION) ==
  Bus Element In2 : Inport  PortName=31X-529P
  Bus Element In1 : Inport  Port=2  PortName=528-529C
  Bus Element Out2 : Outport  PortName=529-522P
  Bus Element Out3 : Outport  Port=2  PortName=529-523P
  Bus Element Out4 : Outport  Port=3  PortName=529-524P
  Bus Element Out5 : Outport  Port=4  PortName=529-528P
  Bus Element Out1 : Outport  Port=5  PortName=529-528C

== system SYSTEM/SHIP/500 (AUXILLIARY SYSTEMS)/52X (FUEL)/52X FUEL/525 (ME FO PIPING)/525 ABSENT ==
  524-525FO : PMIOPort  Side=Right  ConnectionType=Bus: FuelOil_P
  525-520FO : PMIOPort  Port=2  Side=Left  ConnectionType=Bus: FuelOil_P
  525-20XFO : PMIOPort  Port=3  Side=Left  ConnectionType=Bus: FuelOil_P
  20X-525FO : PMIOPort  Port=4  Side=Right  ConnectionType=Bus: FuelOil_P
  525-528C_elem : Outport  PortName=525-528C

== system SYSTEM/SHIP/500 (AUXILLIARY SYSTEMS)/52X (FUEL)/52X FUEL/525 (ME FO PIPING)/525 ME FO PIPING ==
  524-525FO : PMIOPort  Side=Right  ConnectionType=Bus: FuelOil_P
  525-520FO : PMIOPort  Port=2  Side=Left  ConnectionType=Bus: FuelOil_P
  525-20XFO : PMIOPort  Port=3  Side=Left  ConnectionType=Bus: FuelOil_P
  20X-525FO : PMIOPort  Port=4  Side=Right  ConnectionType=Bus: FuelOil_P
  Bus Element Out1 : Outport  PortName=525-528C

== system SYSTEM/SHIP/500 (AUXILLIARY SYSTEMS)/52X (FUEL)/52X FUEL/526 (GS FO PIPING)/526 ABSENT ==
  524-526FO : PMIOPort  Side=Right  ConnectionType=Bus: FuelOil_P
  526-520FO : PMIOPort  Port=2  Side=Left  ConnectionType=Bus: FuelOil_P
  526-30XFO : PMIOPort  Port=3  Side=Left  ConnectionType=Bus: FuelOil_P
  30X-526FO : PMIOPort  Port=4  Side=Right  ConnectionType=Bus: FuelOil_P
  526-528C_elem : Outport  PortName=526-528C

== system SYSTEM/SHIP/500 (AUXILLIARY SYSTEMS)/52X (FUEL)/52X FUEL/526 (GS FO PIPING)/526 GS FO PIPING ==
  524-526FO : PMIOPort  Side=Right  ConnectionType=Bus: FuelOil_P
  526-520FO : PMIOPort  Port=2  Side=Left  ConnectionType=Bus: FuelOil_P
  526-30XFO : PMIOPort  Port=3  Side=Left  ConnectionType=Bus: FuelOil_P
  30X-526FO : PMIOPort  Port=4  Side=Right  ConnectionType=Bus: FuelOil_P
  Bus Element Out1 : Outport  PortName=526-528C

== system SYSTEM/SHIP/500 (AUXILLIARY SYSTEMS)/52X (FUEL)/52X FUEL/527 (MISSION FO PIPING)/527 ABSENT ==
  524-527FO : PMIOPort  Side=Right  ConnectionType=Bus: FuelOil_P
  527-520FO : PMIOPort  Port=2  Side=Left  ConnectionType=Bus: FuelOil_P
  527-55XFO : PMIOPort  Port=3  Side=Left  ConnectionType=Bus: FuelOil_P
  55X-527FO : PMIOPort  Port=4  Side=Right  ConnectionType=Bus: FuelOil_P
  527-528C_elem : Outport  PortName=527-528C

== system SYSTEM/SHIP/500 (AUXILLIARY SYSTEMS)/52X (FUEL)/52X FUEL/527 (MISSION FO PIPING)/527 MISSION FO PIPING ==
  524-527FO : PMIOPort  Side=Right  ConnectionType=Bus: FuelOil_P
  527-520FO : PMIOPort  Port=2  Side=Left  ConnectionType=Bus: FuelOil_P
  527-55XFO : PMIOPort  Port=3  Side=Left  ConnectionType=Bus: FuelOil_P
  55X-527FO : PMIOPort  Port=4  Side=Right  ConnectionType=Bus: FuelOil_P
  Bus Element Out1 : Outport  PortName=527-528C
